simulink model "h2o"  (R2018a)
settings: Solver=FixedStepAuto  StartTime=0.0  StopTime=10.0  RelTol=1e-3
model workspace (MAT data in the model file):
  jumpingImg = [255 255 255 255 255 255 255 255 255 255 255 255 ... (960000 elements, 800x400x3)]
  runningImg = [255 255 255 255 255 255 255 255 255 255 255 255 ... (960000 elements, 800x400x3)]
  sittingImg = [255 255 255 255 255 255 255 255 255 255 255 255 ... (960000 elements, 800x400x3)]
  standingImg = [255 255 255 255 255 255 255 255 255 255 255 255 ... (960000 elements, 800x400x3)]
  walkingImg = [255 255 255 255 255 255 255 255 255 255 255 255 ... (960000 elements, 800x400x3)]
undefined symbols (not defined in the file or in its folder): Acc_X, Acc_Y, Acc_Z, Predicted_Activity, slexHARAndroidExample
libraries: androiduilib x4, androidsensorlib x1
(part 1 of 2)
settings Model: Creator=The MathWorks, Inc.  LastModifiedBy=bobch
settings SolverCC: DecoupledContinuousIntegration=on
settings OptimizationCC: EnhancedBackFolding=on  StrengthReduction=on  PassReuseOutputArgsThreshold=0  MaxStackSize=64  OptimizeBlockOrder=speed  DifferentSizesBufferReuse=on
settings DebuggingCC: ParameterTunabilityLossMsg=error
settings HardwareCC: ProdBitPerPointer=32  ProdBitPerSizeT=32  ProdBitPerPtrDiffT=32  ProdLargestAtomicInteger=Long  ProdLargestAtomicFloat=Double  ProdWordSize=32  ProdHWDeviceType=ARM Compatible->ARM Cortex  UseEmbeddedCoderFeatures=off  UseSimulinkCoderFeatures=off
settings SFSimCC: MATLABDynamicMemAlloc=off
settings RTWCC: SystemTargetFile=ert.tlc  HardwareBoard=Android Device  TLCOptions="-aInlineSetEventsForThisBaseRateFcn=TLC_FALSE -aSuppressMultiTaskScheduler=TLC_FALSE  -aRateBasedStepFcn=0"  TemplateMakefile=ert_default_tmf  GenerateReport=on  Toolchain=Android SDK/NDK Tools  BuildConfiguration=Faster Runs  LaunchReport=on
settings CodeAppCC: ForceParamTrailComments=on  OperatorAnnotations=on
settings ERTTargetCC: ERTCustomFileBanners=off  SupportContinuousTime=on  SupportNonInlinedSFcns=on  RemoveResetFunc=off  SupportVariableSizeSignals=on  ModelStepFunctionPrototypeControlCompliant=off

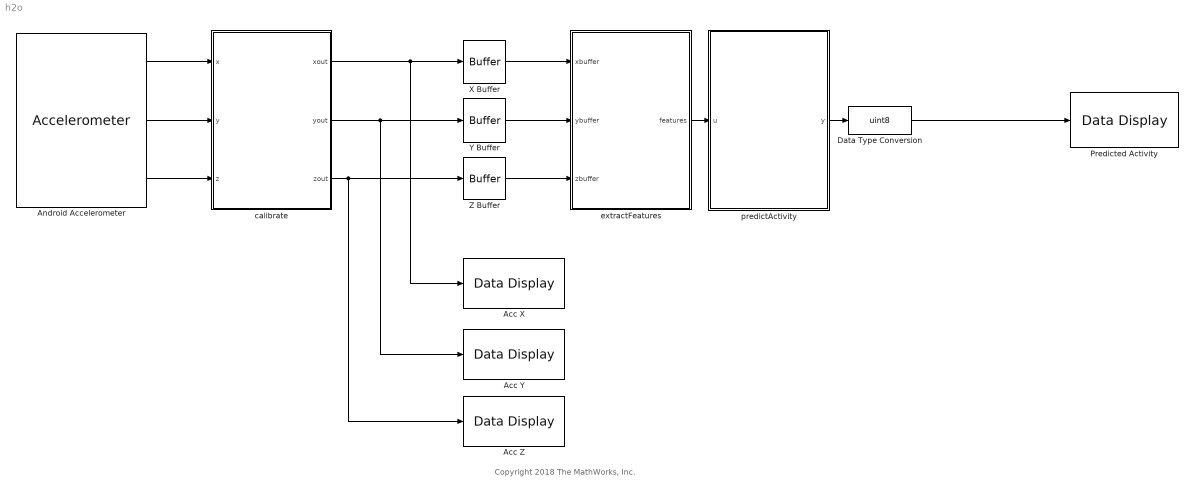
== system h2o ==
  note: Copyright 2018 The MathWorks, Inc.
  Acc X : androiduilib/Data Display  DataDisplayId=slexHARAndroidExample/Acc_X  Format=Float  Precision=6  SimulateUsing=Code generation  blockPlatform=Android
      settings: SourceProductName=Simulink Support Package for Android Devices  SourceProductBaseCode=ANDROID
  Acc Y : androiduilib/Data Display  DataDisplayId=slexHARAndroidExample/Acc_Y  Format=Float  Precision=6  SimulateUsing=Code generation  blockPlatform=Android
      settings: SourceProductName=Simulink Support Package for Android Devices  SourceProductBaseCode=ANDROID
  Acc Z : androiduilib/Data Display  DataDisplayId=slexHARAndroidExample/Acc_Z  Format=Float  Precision=6  SimulateUsing=Code generation  blockPlatform=Android
      settings: SourceProductName=Simulink Support Package for Android Devices  SourceProductBaseCode=ANDROID
  Android Accelerometer : androidsensorlib/Accelerometer  OutputVector=off  SampleTime=0.1  BlockPlatform=Android
      settings: SourceProductName=Simulink Support Package for Android Devices  SourceProductBaseCode=ANDROID
  Data Type Conversion : DataTypeConversion  OutDataTypeStr=uint8
  Predicted Activity : androiduilib/Data Display  DataDisplayId=slexHARAndroidExample/Predicted_Activity  Format=Float  Precision=6  SimulateUsing=Code generation  blockPlatform=Android
      settings: SourceProductName=Simulink Support Package for Android Devices  SourceProductBaseCode=ANDROID
  X Buffer : Buffer  N=32  V=12  OutputFrames=off
  Y Buffer : Buffer  N=32  V=12  OutputFrames=off
  Z Buffer : Buffer  N=32  V=12  OutputFrames=off
  calibrate : MATLAB Function  TreatAsAtomicUnit=on
  extractFeatures : MATLAB Function  TreatAsAtomicUnit=on
  predictActivity : MATLAB Function  TreatAsAtomicUnit=on
  wires:
  Data Type Conversion/1 -> Predicted Activity/1
  calibrate/3(zout) -> Acc Z/1, Z Buffer/1
  Y Buffer/1 -> extractFeatures/2(ybuffer)
  Android Accelerometer/2 -> calibrate/2(y)
  extractFeatures/1(features) -> predictActivity/1(u)
  X Buffer/1 -> extractFeatures/1(xbuffer)
  Android Accelerometer/3 -> calibrate/3(z)
  calibrate/2(yout) -> Acc Y/1, Y Buffer/1
  predictActivity/1(y) -> Data Type Conversion/1
  Z Buffer/1 -> extractFeatures/3(zbuffer)
  calibrate/1(xout) -> Acc X/1, X Buffer/1
  Android Accelerometer/1 -> calibrate/1(x)
